simulink model "IA331_Rubtsov_Lab9"  (R2023b)
settings: Solver=VariableStepAuto  StartTime=0.0  StopTime=200  RelTol=1e-3
model workspace (MAT data in the model file):
  Queries_MAX = 100
  Task_Weight = 2
  Threshold_Val = 0.1
  lambda = 0.25
values from neighbouring files (symbols this model uses):
  m = 200    [IA331_Rubtsov_Lab1_3.m]    (also in IA331_Rubtsov_Lab4.m = 10; IA331_Rubtsov_Lab5.m = 1)
  n = length(x)    [IA331_Rubtsov_Lab2.m]    (also in IA331_Rubtsov_Lab3_2.m = sample_points(i); IA331_Rubtsov_Lab3_3.m = n_vals(i); IA331_Rubtsov_Lab4.m = 10)
settings Model: Creator=error  LastModifiedBy=error

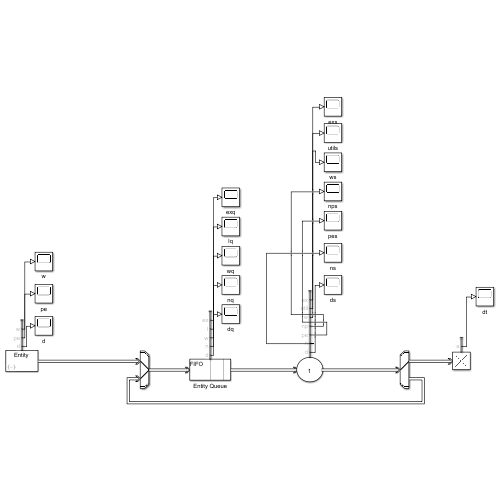
[thumbnail: Simulink's stored preview of the top-level diagram]
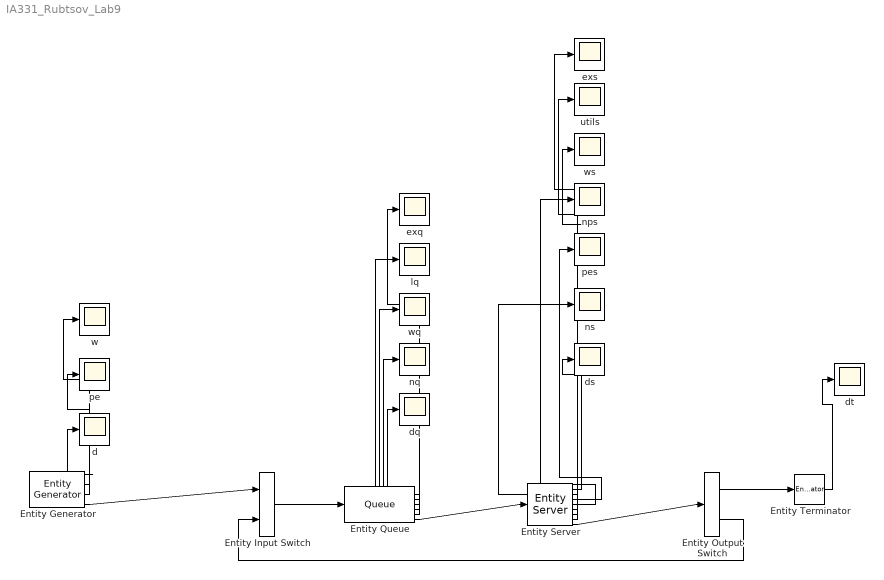
== system IA331_Rubtsov_Lab9 ==
  Entity Input Switch : EntityInputSwitch  InputPortMessageModes=m,m  OutputPortMessageModes=m
  Entity Output Switch : EntityOutputSwitch  InputPortMessageModes=m  OutputPortMessageModes=m,m  SwitchingCriterion=From attribute  SwitchAttributeName=reject
  Entity Generator : EntityGenerator  OutputPortMessageModes=n,n,n,m  TimeSource=MATLAB action  IntergenerationTimeAction=|  GenerateAction=entity.reject = randi([1, 2]);  AttributeName=weight|reject  AttributeInitialValue=1|1  NumberEntitiesDeparted=on  PendingEntityInBlock=on  AverageIntergenerationTime=on  EntityType=Structured  EntityTypeName=Entity
      | persistent n;
      | if isempty(n)
      |     n = 0;
      | end
      | n = n + 1;
      | 
      | if n <= Queries_MAX
      |     dt = exprnd(1/lambda);
      | else
      |     dt = inf;
      | end
      settings: OutputPortMap=o0,o1,o2,o3
  Entity Queue : Queue  InputPortMessageModes=m  OutputPortMessageModes=n,n,n,n,n,m  NumberEntitiesDeparted=on  NumEntitiesExtracted=on  NumberEntitiesInBlock=on  AverageWait=on  AverageQueueLength=on
      settings: OutputPortMap=o0,o1,o2,o3,o7,o5
  Entity Server : EntityServer  InputPortMessageModes=m  OutputPortMessageModes=n,n,n,n,n,n,n,m  Capacity=1  ServiceTimeSource=MATLAB action  ServiceTimeAction=dt = rand(1,1) + entity.weight;  NumberEntitiesDeparted=on  NumberEntitiesInBlock=on  PendingEntityPresentInBlock=on  NumberEntitiesPending=on  AverageWait=on  Utilization=on  NumEntitiesExtracted=on
      settings: OutputPortMap=o0,o1,o2,o3,o4,o5,o12,o9
  Entity Terminator : EntityTerminator  InputPortMessageModes=m  NumberEntitiesArrived=on
      settings: OutputPortMap=o0
  d : Scope
  dq : Scope
  ds : Scope
  dt : Scope
  exq : Scope
  exs : Scope
  lq : Scope
  nps : Scope
  nq : Scope
  ns : Scope
  pe : Scope
  pes : Scope
  utils : Scope
  w : Scope
  wq : Scope
  ws : Scope
  wires:
  Entity Generator/4 -> Entity Input Switch/1
  Entity Input Switch/1 -> Entity Queue/1
  Entity Queue/6 -> Entity Server/1
  Entity Server/8 -> Entity Output Switch/1
  Entity Output Switch/2 -> Entity Input Switch/2
  Entity Output Switch/1 -> Entity Terminator/1
  Entity Terminator/1 -> dt/1
  Entity Generator/1 -> d/1
  Entity Generator/2 -> pe/1
  Entity Generator/3 -> w/1
  Entity Queue/1 -> dq/1
  Entity Queue/2 -> nq/1
  Entity Queue/3 -> wq/1
  Entity Queue/4 -> lq/1
  Entity Queue/5 -> exq/1
  Entity Server/1 -> ds/1
  Entity Server/2 -> ns/1
  Entity Server/3 -> pes/1
  Entity Server/4 -> nps/1
  Entity Server/5 -> ws/1
  Entity Server/6 -> utils/1
  Entity Server/7 -> exs/1
